simulink model "untitled"  (R2015a)
settings: Solver=ode45  StartTime=0.0  StopTime=1000  RelTol=1e-3
settings Model: Creator=Diogo  LastModifiedBy=Diogo

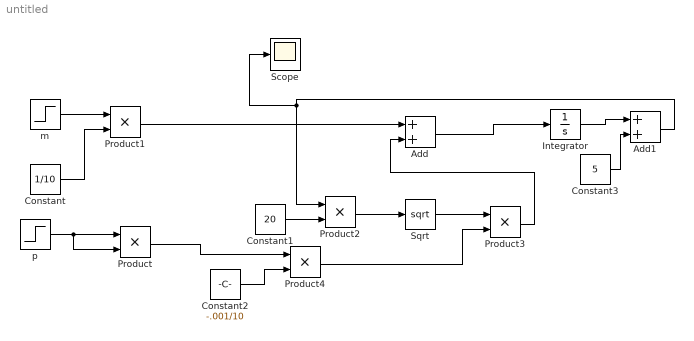
== system untitled ==
  Add : Sum
  Add1 : Sum
  Constant : Constant  Value=1/10
  Constant1 : Constant  Value=20
  Constant2 : Constant  Value=-.001/10
  Constant3 : Constant  Value=5
  Integrator : Integrator
  Product{,1..4} (5 alike) : Product
  Scope : Scope
  Sqrt : Sqrt  SaturateOnIntegerOverflow=on
  m : Step  Before=1  After=2  SampleTime=0
  p : Step  Before=10  After=10  SampleTime=0
  wires:
  m/1 -> Product1/1
  Constant/1 -> Product1/2
  p/1 -> Product/2, Product/1
  Constant1/1 -> Product2/2
  Add1/1 -> Scope/1, Product2/1
  Product2/1 -> Sqrt/1
  Sqrt/1 -> Product3/1
  Product/1 -> Product4/1
  Constant2/1 -> Product4/2
  Product4/1 -> Product3/2
  Product3/1 -> Add/2
  Product1/1 -> Add/1
  Add/1 -> Integrator/1
  Integrator/1 -> Add1/1
  Constant3/1 -> Add1/2
